simulink model "digital_PLL_r2012b"  (Simulink 10.1)
settings: Solver=ode23t  StartTime=0.0  StopTime=1  MaxStep=1e-4  RelTol=1e-4  EnableMultiTasking=on
undefined symbols (not defined in the file or in its folder): DigPLLfun
settings Model: Creator=Wassinger  LastModifiedBy=marco
settings DataIOCC: LimitDataPoints=on  SignalLoggingSaveFormat=ModelDataLogs
settings OptimizationCC: ExpressionDepthLimit=2147483647
settings DebuggingCC: SolverPrmCheckMsg=warning  FcnCallInpInsideContextMsg=warning  StateNameClashWarn=warning

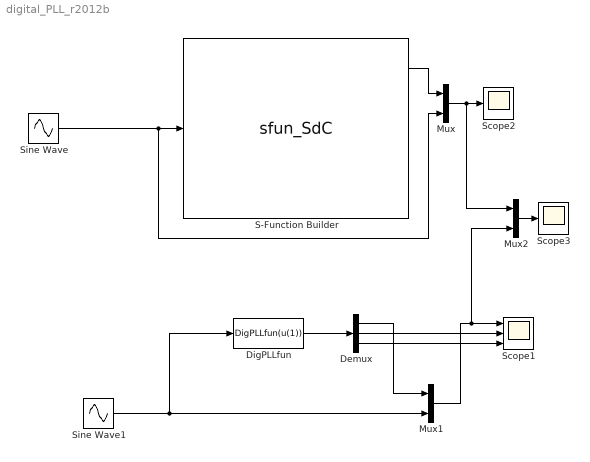
== system digital_PLL_r2012b ==
  Demux : Demux  Outputs=3
  DigPLLfun : MATLABFcn  MATLABFcn=DigPLLfun(u(1))  OutputDimensions=3  SampleTime=1e-3
  Mux : Mux  Inputs=2
  Mux1 : Mux  Inputs=2
  Mux2 : Mux  Inputs=2
  S-Function Builder : S-Function  InitFcn=try, set_param(gcb,'FunctionName','sfun_SdC'), end  FunctionName=sfun_SdC  SFunctionModules=sfun_SdC_wrapper  WizardData=DataTag0  SFunctionDeploymentMode=off  EnableBusSupport=off  mask(S-Function Builder){}
      mask help: The S-Function Builder block creates a wrapper C-MEX S-function from your supplied C code with multiple input ports, output ports, and a variable number of scalar, vector, or matrix parameters. The input and output ports can propagate Simulink built-in data types, fixed-point datatypes, complex, frame, 1-D, and 2-D signals. This block also supports discrete and continuous states of type real. You can optionally have the block generate a TLC file to be used with Real-Time Workshop for code generation.
      mask init:
      | val = [[.9  0.75 0.75 1 1 .9 .9 1]',[1 1 0.75 0.75 .9 .9 1 .9]'];try , sys = get_param(gcb,'SfunBuilderFcnName');if isempty(sys), sys = get_param(gcb,'FunctionName'); end,catch, sys = get_param(gcb,'FunctionName'); end
      settings: CopyFcn=set_param(gcbh,'LinkStatus','none')  PreSaveFcn=try, set_param(gcb,'FunctionName','sfun_SdC'), end  OpenFcn=sfunctionwizard(gcbh)
      mask Display: plot(val(:,1),val(:,2)),disp(sys), port_label('input',1,'Input10V'), port_label('output',1,'Output3_3V'), port_label('output',2,'UserLED'), port_label('output',3,'UserGPIO')
  Scope1 : Scope  NumInputPorts=3
  Scope2 : Scope
  Scope3 : Scope
  Sine Wave : Sin  Amplitude=5  Bias=5  Frequency=50*2*pi  SampleTime=0
  Sine Wave1 : Sin  Amplitude=5  Bias=5  Frequency=50*2*pi  SampleTime=0
  wires:
  S-Function Builder/1 -> Mux/1
  Sine Wave/1 -> S-Function Builder/1, Mux/2
  Mux/1 -> Mux2/1, Scope2/1
  Sine Wave1/1 -> DigPLLfun/1, Mux1/2
  DigPLLfun/1 -> Demux/1
  Mux1/1 -> Mux2/2, Scope1/1
  Demux/1 -> Mux1/1
  Demux/2 -> Scope1/2
  Demux/3 -> Scope1/3
  Mux2/1 -> Scope3/1
